simulink model "sv_power_control_subsystem_final"  (R2023b)
settings: Solver=FixedStepAuto  StartTime=0  StopTime=1  FixedStep=1/5e4/60  MaxStep=1e-4  RelTol=1e-4
StartFcn:
  | tic
StopFcn:
  | toc
undefined symbols (not defined in the file): Ion, Lithium
libraries: spsBatteryLib x30, simulink x30, spsIdealSwitchLib x30, spsSeriesRLCBranchLib x2, spsControlledCurrentSourceLib x1, spsGroundLib x1, spsTriangleGeneratorLib x1, spsVoltageMeasurementLib x1, spspowerguiLib x1
settings Model: SimulationMode=accelerator  Creator=The MathWorks, Inc.  LastModifiedBy=zhaoxu
settings SolverCC: ZeroCrossAlgorithm=Adaptive  AlgebraicLoopSolver=TrustRegion  AutoInsertRateTranBlk=on
settings DataIOCC: LimitDataPoints=on  SaveFormat=Array  SaveOutput=off  SignalLogging=off  SaveTime=off  ReturnWorkspaceOutputs=off
settings OptimizationCC: ExpressionDepthLimit=2147483647  LifeSpan=inf
settings DebuggingCC: UnderspecifiedInitializationDetection=Classic  MergeDetectMultiDrivingBlocksExec=none  IgnoredZcDiagnostic=none  SolverPrmCheckMsg=warning  MultiTaskRateTransMsg=warning  FcnCallInpInsideContextMsg=warning  UnconnectedInputMsg=warning  UnconnectedOutputMsg=warning  UnconnectedLineMsg=warning  StateNameClashWarn=warning  SFUnexpectedBacktrackingDiag=warning  SFNoUnconditionalDefaultTransitionDiag=warning  SFExecutionAtInitializationDiag=none  ArithmeticOperatorsInVariantConditions=warning
settings HardwareCC: ProdHWDeviceType=AMD->x86-64 (Windows64)
settings ModelReferenceCC: EnableRefExpFcnMdlSchedulingChecks=on  PropagateSignalLabelsOutOfModel=off
settings SFSimCC: SimUseLocalCustomCode=off  CustomCodeUndefinedFunction=UseInterfaceOnly  SimTargetLang=C++
settings RTWCC: RTWUseLocalCustomCode=off  DLArmComputeVersion=19.05
settings CodeAppCC: StateflowObjectComments=on
settings GRTTargetCC: TargetLangStandard=C89/C90 (ANSI)  CombineOutputUpdateFcns=off  GRTInterface=on
settings ConfigComp: CovMetricSettings=dw  CovSaveCumulativeToWorkspaceVar=on  CovSaveSingleToWorkspaceVar=on  CovExternalEMLEnable=off  CovSFcnEnable=off
settings SimscapeCC: SimscapeNormalizeSystem=off  SimscapeNominalValues={1, 'bar'; 1, 'cm^3/s'; 1, 'bar*kg/s'; 1, 'kJ/kg'; 1, 'kW'; }

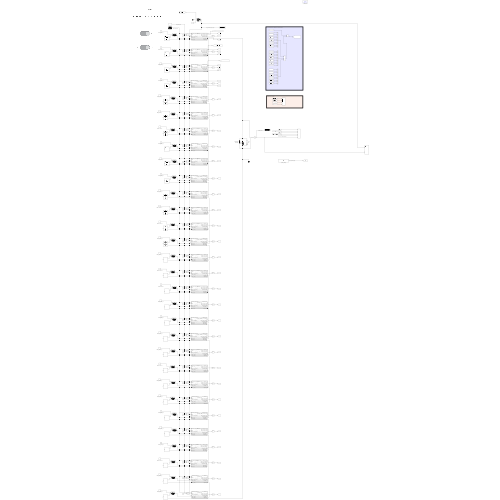
[thumbnail: Simulink's stored preview of the top-level diagram]
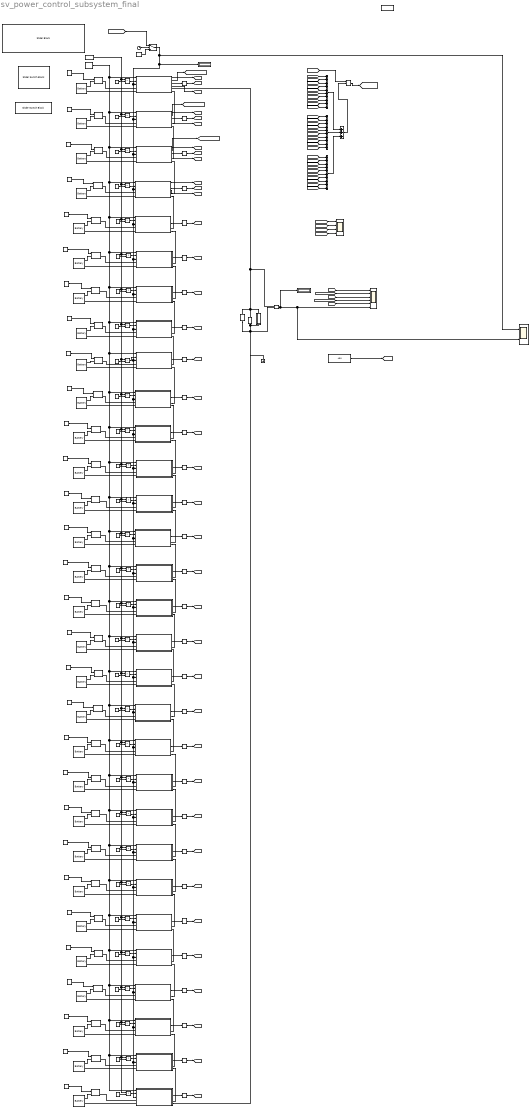
== system sv_power_control_subsystem_final ==
  note: Synchronous_PWM
  note: The average given voltage for each module
  Add1 : Sum  Inputs=+++
  Add2 : Sum  Inputs=++++++++++
  Add3 : Sum  Inputs=++++++++++
  Add4 : Sum  Inputs=++++++++++
  Battery{1..30} (30 alike) : spsBatteryLib/Battery  BatType=Lithium-Ion  ShowTempParam=off  ThermalPreset=no  ShowAgeParam=off  NomV=25.6  NomQ=50  SOC=70  Batt_Tr=30  PresetModel=on  MaxQ=50  MinV=19.2  FullV=29.7981  Dis_rate=21.7391  R=0.00512  Normal_OP=45.2174  expZone="[27.6579      2.45652]"  current=[6.5 13 32.5]  Units=Ampere-hour  Tci=20  NomT=20  T2=-30  MaxQ2=4.8  FullV2=7.1  Normal_OP2=5.655  expZone2="[6.58           1]"  Rca=0.6  ti=2000  Dp=0  Neq0=0  Tsim=1e6  Ta1=25  Qeol=5.4*0.9  Reol=0.013333*1.2  Char_age=[2.3478, 3]  Dis_age=[2.3478, 10]  N1=1500  N2=10500  N3=1000  N4=1400  Ta2=45  N5=950
  Battery_Enable_{1..30} (30 alike) : Constant
  Clock : Clock
  Compare To Constant{,1..29} (30 alike) : simulink/Logic and Bit Operations/Compare To Constant  relop=>=  const=15  OutDataTypeStr=uint8
  Constant : Constant  Value=10
  Constant1 : Constant  Value=0
  Constant10 : Constant  Value=8
  Constant11 : Constant  Value=9
  Constant12 : Constant  Value=10
  Constant13 : Constant  Value=11
  Constant14 : Constant  Value=12
  Constant15 : Constant  Value=17
  Constant16 : Constant  Value=18
  Constant17 : Constant  Value=19
  Constant18 : Constant  Value=20
  Constant19 : Constant  Value=21
  Constant2 : Constant
  Constant20 : Constant  Value=13
  Constant21 : Constant  Value=14
  Constant22 : Constant  Value=15
  Constant23 : Constant  Value=16
  Constant24 : Constant  Value=25
  Constant25 : Constant  Value=26
  Constant26 : Constant  Value=27
  Constant27 : Constant  Value=28
  Constant28 : Constant  Value=29
  Constant29 : Constant  Value=22
  Constant3 : Constant  Value=2
  Constant30 : Constant  Value=23
  Constant31 : Constant  Value=24
  Constant4 : Constant  Value=3
  Constant5 : Constant  Value=4
  Constant6 : Constant  Value=5
  Constant7 : Constant  Value=1/5e4/30
  Constant8 : Constant  Value=6
  Constant9 : Constant  Value=7
  Cyclic load : Subsystem
  Display : Display
  Display2 : Display
  Divide : Product  Inputs=*/
  Fixed load : spsSeriesRLCBranchLib/Series RLC Branch  LConnTagsString=__new0  RConnTagsString=__new0  BranchType=R  Resistance=3.75  Inductance=1e-3  SetiL0=off  InitialCurrent=0  Capacitance=1e-6  Setx0=off  InitialVoltage=0  Measurements=None
  Ground : spsGroundLib/Ground  LConnTagsString=a
  Ideal Switch{,1..29} (30 alike) : spsIdealSwitchLib/Ideal Switch  Ron=0.001  Lon=0  IC=0  Rs=1e5  Cs=inf  Measurements=on
  Product{,1..29} (30 alike) : Product
  Scope : Scope  NumInputPorts=6
  Scope2 : Scope  NumInputPorts=4
  Scope3 : Scope  NumInputPorts=2
  Slider : SliderBlock  ScaleMin=400  ScaleMax=768
  Slider Switch : SliderSwitchBlock
      settings: Values={{'Off', 'On'}, [0 1]}
  Slider Switch1 : SliderSwitchBlock
      settings: Values={{'Off', 'On'}, [0 1]}
  Smoothing capacitor : spsSeriesRLCBranchLib/Series RLC Branch  LConnTagsString=__new0  RConnTagsString=__new0  BranchType=C  Resistance=1  Inductance=1e-3  SetiL0=off  InitialCurrent=0  Capacitance=1.6e-5  Setx0=off  InitialVoltage=0  Measurements=None
  Subsystem{,1..29} (30 alike) : Subsystem  ReferencedSubsystem=Subsystem_final
  Switch : Switch  Criteria=u2 > Threshold  Threshold=0.001  SaturateOnIntegerOverflow=off  InputSameDT=off
  System_Voltage : Constant  Value=450
  Triangle Generator : spsTriangleGeneratorLib/Triangle Generator  Freq=50000  Phase=0  Ts=0
  Voltage Measurement : spsVoltageMeasurementLib/Voltage Measurement  PhasorSimulation=off  OutputType=Complex  PSBequivalent=0
  powergui : spspowerguiLib/powergui  Priority=1  SimulationMode=Discrete  SampleTime=1/5e4/60  frequency=60  Iterations=50  frequencyindice=0  Pbase=100e6  ErrMax=1e-4  UnitsV=kV  UnitsW=MW  buscounter=0  FunctionMessages=off  echomessages=off  EnableUseOfTLC=off  CurrentSourceSwitches=off  DisableSnubberDevices=off  DisableRonSwitches=off  DisableVfSwitches=off  DisplayEquations=off  AutomaticDiscreteSolvers=off  SolverType=Tustin/Backward Euler (TBE)  Interpol=off  ExternalGateDelay=off  methode=off  Ts=100  x0status=blocks  SPID=on  SwTol=0  HookPort=off  NonlinearTolerance=1e-4  nMaxIteration=100  ContinueOnMaxIteration=off  RestoreLinks=warning  ResistiveCurrentMeasurement=off  Frange=[0:2:500]  Ylog=off  Xlog=on  ShowGrid=off  save=off  variable=ZData  structure=0  ZoomFFT=on  StartTime=0.0  cycles=1  DisplayStyle=1  fundamental=60  FreqAxis=off  MaxFrequency=1000  frequencyindicesteady=1  RmsSteady=1  display=off
  wires:
  Battery_Enable_1/1 -> Ideal Switch/1
  Battery_Enable_2/1 -> Ideal Switch1/1
  Battery_Enable_3/1 -> Ideal Switch2/1
  Battery_Enable_4/1 -> Ideal Switch3/1
  Battery_Enable_5/1 -> Ideal Switch4/1
  Battery_Enable_7/1 -> Ideal Switch6/1
  Battery_Enable_6/1 -> Ideal Switch5/1
  Subsystem1/3 -> Compare To Constant2/1
  Subsystem2/3 -> Compare To Constant3/1
  Subsystem4/3 -> Compare To Constant1/1
  Add1/1 -> Divide/2
  Subsystem/3 -> Compare To Constant/1
  Subsystem6/3 -> Compare To Constant4/1
  Subsystem3/3 -> Compare To Constant5/1
  Subsystem5/3 -> Compare To Constant6/1
  Product/1 -> Subsystem/2
  Product1/1 -> Subsystem4/2
  Product2/1 -> Subsystem1/2
  Product3/1 -> Subsystem2/2
  Product4/1 -> Subsystem6/2
  Product5/1 -> Subsystem3/2
  Product6/1 -> Subsystem5/2
  Constant1/1 -> Product/2
  Constant2/1 -> Product1/2
  Constant3/1 -> Product2/2
  Constant4/1 -> Product3/2
  Constant5/1 -> Product4/2
  Constant6/1 -> Product5/2
  Constant8/1 -> Product6/2
  Constant/1 -> Switch/3
  Clock/1 -> Switch/2
  [control_V] -> Divide/1
  Subsystem/1 -> [CV1]  "CV1"
  [CV1] -> Scope/1
  [Battery_Current_1] -> Scope/2
  [Battery_Current_2] -> Scope/4
  Subsystem4/1 -> [CV2]  "CV2"
  Subsystem1/1 -> [CV3]  "CV3"
  Subsystem2/1 -> [CV4]  "CV4"
  [CV2] -> Scope/3
  [i_load] -> Scope/5  "yclic load current"
  Compare To Constant/1 -> [BV1]
  Compare To Constant1/1 -> [BV2]
  Compare To Constant2/1 -> [BV3]
  Compare To Constant3/1 -> [BV4]
  Compare To Constant4/1 -> [BV5]
  Compare To Constant5/1 -> [BV6]
  Compare To Constant6/1 -> [BV7]
  Divide/1 -> [Average_voltage]
  [Average_voltage] -> Switch/1
  Subsystem/4 -> [S_PWM1]
  Subsystem4/4 -> [S_PWM2]
  Subsystem1/4 -> [S_PWM3]
  Subsystem2/4 -> [S_PWM4]
  [S_PWM1] -> Scope2/1
  [S_PWM2] -> Scope2/2
  [S_PWM3] -> Scope2/3
  [S_PWM4] -> Scope2/4
  Voltage Measurement/1 -> Scope3/2, Scope/6, Display2/1  "HV_BUS_Voltage"
  Product9/1 -> Subsystem8/2
  Constant14/1 -> Product12/2
  Constant12/1 -> Product10/2
  Constant9/1 -> Product7/2
  Compare To Constant9/1 -> [BV10]
  Subsystem10/3 -> Compare To Constant7/1
  Compare To Constant12/1 -> [BV13]
  Subsystem12/3 -> Compare To Constant10/1
  Battery_Enable_8/1 -> Ideal Switch7/1
  Compare To Constant8/1 -> [BV9]
  Constant13/1 -> Product11/2
  Compare To Constant10/1 -> [BV11]
  Battery_Enable_12/1 -> Ideal Switch11/1
  Product12/1 -> Subsystem11/2
  Subsystem11/3 -> Compare To Constant12/1
  Product8/1 -> Subsystem7/2
  Subsystem8/3 -> Compare To Constant9/1
  Subsystem7/3 -> Compare To Constant8/1
  Product7/1 -> Subsystem10/2
  Product11/1 -> Subsystem9/2
  Battery_Enable_11/1 -> Ideal Switch10/1
  Constant10/1 -> Product8/2
  Constant11/1 -> Product9/2
  Battery_Enable_13/1 -> Ideal Switch12/1
  Compare To Constant7/1 -> [BV8]
  Compare To Constant11/1 -> [BV12]
  Product10/1 -> Subsystem12/2
  Battery_Enable_9/1 -> Ideal Switch8/1
  Subsystem9/3 -> Compare To Constant11/1
  Battery_Enable_10/1 -> Ideal Switch9/1
  Constant16/1 -> Product21/2
  Product13/1 -> Subsystem15/2
  Constant15/1 -> Product20/2
  Compare To Constant19/1 -> [BV17]
  Battery_Enable_14/1 -> Ideal Switch21/1
  Battery_Enable_17/1 -> Ideal Switch15/1
  Product14/1 -> Subsystem21/2
  Battery_Enable_22/1 -> Ideal Switch20/1
  Subsystem21/3 -> Compare To Constant14/1
  Battery_Enable_15/1 -> Ideal Switch13/1
  Product15/1 -> Subsystem14/2
  Subsystem14/3 -> Compare To Constant15/1
  Product19/1 -> Subsystem13/2
  Constant18/1 -> Product14/2
  Compare To Constant14/1 -> [BV21]
  Product20/1 -> Subsystem19/2
  Subsystem19/3 -> Compare To Constant20/1
  Compare To Constant13/1 -> [BV20]
  Compare To Constant20/1 -> [BV18]
  Compare To Constant15/1 -> [BV22]
  Subsystem15/3 -> Compare To Constant13/1
  Battery_Enable_16/1 -> Ideal Switch14/1
  Constant17/1 -> Product13/2
  Compare To Constant21/1 -> [BV19]
  Constant19/1 -> Product15/2
  Product21/1 -> Subsystem20/2
  Constant23/1 -> Product19/2
  Subsystem20/3 -> Compare To Constant21/1
  Subsystem13/3 -> Compare To Constant19/1
  Constant20/1 -> Product16/2
  Compare To Constant18/1 -> [BV16]
  Subsystem18/3 -> Compare To Constant16/1
  Constant21/1 -> Product17/2
  Product16/1 -> Subsystem18/2
  Battery_Enable_21/1 -> Ideal Switch19/1
  Compare To Constant16/1 -> [BV14]
  Constant22/1 -> Product18/2
  Battery_Enable_19/1 -> Ideal Switch17/1
  Product18/1 -> Subsystem17/2
  Subsystem17/3 -> Compare To Constant18/1
  Product17/1 -> Subsystem16/2
  Subsystem16/3 -> Compare To Constant17/1
  Battery_Enable_18/1 -> Ideal Switch16/1
  Battery_Enable_20/1 -> Ideal Switch18/1
  Compare To Constant17/1 -> [BV15]
  Constant7/1 -> Product4/1, Product5/1, Product10/1, Product11/1, Product16/1, Product17/1, Product13/1, Product14/1, Product25/1, Product22/1, Product23/1, Product24/1, Product29/1, Product28/1, Product27/1, Product26/1, Product15/1, Product21/1, Product20/1, Product19/1, Product18/1, Product12/1, Product9/1, Product8/1, Product7/1, Product6/1, Product3/1, Product2/1, Product1/1, Product/1  "PWM_Phase_Base"
  Battery_Enable_28/1 -> Ideal Switch26/1
  Product25/1 -> Subsystem25/2
  Subsystem25/3 -> Compare To Constant25/1
  Compare To Constant25/1 -> [BV23]
  Subsystem26/3 -> Compare To Constant26/1
  Triangle Generator/1 -> Subsystem/1, Subsystem4/1, Subsystem1/1, Subsystem2/1, Subsystem6/1, Subsystem3/1, Subsystem10/1, Subsystem8/1, Subsystem12/1, Subsystem9/1, Subsystem18/1, Subsystem16/1, Subsystem13/1, Subsystem19/1, Subsystem20/1, Subsystem15/1, Subsystem21/1, Subsystem25/1, Subsystem22/1, Subsystem27/1, Subsystem28/1, Subsystem24/1, Subsystem29/1, Subsystem23/1, Subsystem26/1, Subsystem14/1, Subsystem17/1, Subsystem11/1, Subsystem7/1, Subsystem5/1  "PWM_Ref_Signal"
  Battery_Enable_27/1 -> Ideal Switch25/1
  Product26/1 -> Subsystem26/2
  Battery_Enable_29/1 -> Ideal Switch27/1
  Compare To Constant26/1 -> [BV24]
  Subsystem22/3 -> Compare To Constant27/1
  Subsystem28/3 -> Compare To Constant29/1
  Product29/1 -> Subsystem28/2
  Compare To Constant29/1 -> [BV27]
  Compare To Constant28/1 -> [BV26]
  Battery_Enable_30/1 -> Ideal Switch28/1
  Product27/1 -> Subsystem22/2
  Battery_Enable_25/1 -> Ideal Switch23/1
  Product23/1 -> Subsystem29/2
  Compare To Constant23/1 -> [BV29]
  Subsystem29/3 -> Compare To Constant23/1
  Battery_Enable_24/1 -> Ideal Switch22/1
  Subsystem23/3 -> Compare To Constant24/1
  Subsystem24/3 -> Compare To Constant22/1
  Constant24/1 -> Product28/2
  Constant26/1 -> Product22/2
  Product22/1 -> Subsystem24/2
  Constant29/1 -> Product25/2
  Battery_Enable_23/1 -> Ideal Switch29/1
  Constant28/1 -> Product24/2
  Product24/1 -> Subsystem23/2
  Constant27/1 -> Product23/2
  Compare To Constant22/1 -> [BV28]
  Battery_Enable_26/1 -> Ideal Switch24/1
  Subsystem27/3 -> Compare To Constant28/1
  Compare To Constant27/1 -> [BV25]
  Compare To Constant24/1 -> [BV30]
  Constant30/1 -> Product26/2
  Constant31/1 -> Product27/2
  Product28/1 -> Subsystem27/2
  Constant25/1 -> Product29/2
  [BV30] -> Add4/10
  [BV21] -> Add4/1
  [BV22] -> Add4/2
  [BV23] -> Add4/3
  [BV24] -> Add4/4
  [BV25] -> Add4/5
  [BV26] -> Add4/6
  [BV27] -> Add4/7
  [BV28] -> Add4/8
  [BV29] -> Add4/9
  [BV11] -> Add3/1
  [BV12] -> Add3/2
  [BV13] -> Add3/3
  [BV14] -> Add3/4
  [BV15] -> Add3/5
  [BV16] -> Add3/6
  [BV17] -> Add3/7
  [BV18] -> Add3/8
  [BV19] -> Add3/9
  [BV20] -> Add3/10
  [BV1] -> Add2/1
  [BV2] -> Add2/2
  [BV3] -> Add2/3
  [BV4] -> Add2/4
  [BV5] -> Add2/5
  [BV6] -> Add2/6
  [BV7] -> Add2/7
  [BV8] -> Add2/8
  [BV9] -> Add2/9
  [BV10] -> Add2/10
  Add4/1 -> Add1/3
  Add3/1 -> Add1/2
  Add2/1 -> Add1/1
  Switch/1 -> Scope3/1, Display/1, Subsystem23/3, Subsystem29/3, Subsystem24/3, Subsystem28/3, Subsystem27/3, Subsystem22/3, Subsystem26/3, Subsystem25/3, Subsystem14/3, Subsystem21/3, Subsystem15/3, Subsystem20/3, Subsystem19/3, Subsystem13/3, Subsystem17/3, Subsystem16/3, Subsystem18/3, Subsystem11/3, Subsystem9/3, Subsystem12/3, Subsystem8/3, Subsystem7/3, Subsystem10/3, Subsystem5/3, Subsystem3/3, Subsystem6/3, Subsystem2/3, Subsystem1/3, Subsystem4/3, Subsystem/3  "Single_Modular_Voltage_Target"
  System_Voltage/1 -> [control_V]  "Target_HV_BUS_Voltage"
  Subsystem/2 -> [Battery_Current_1]
  Subsystem4/2 -> [Battery_Current_2]
  Subsystem1/2 -> [Battery_Current_3]
  connections:
  Ideal Switch/LConn1 -- Battery1/LConn1
  Subsystem/LConn2 -- Battery1/LConn2
  Subsystem/LConn1 -- Ideal Switch/RConn1
  Fixed load/RConn1 -- Ground/LConn1 -- Subsystem23/RConn2 -- Smoothing capacitor/RConn1 -- Voltage Measurement/LConn2 -- Cyclic load/LConn1
  Subsystem4/LConn2 -- Battery2/LConn2
  Ideal Switch1/LConn1 -- Battery2/LConn1
  Subsystem4/LConn1 -- Ideal Switch1/RConn1
  Subsystem4/RConn1 -- Subsystem/RConn2
  Subsystem1/LConn2 -- Battery3/LConn2
  Subsystem1/LConn1 -- Ideal Switch2/RConn1
  Ideal Switch2/LConn1 -- Battery3/LConn1
  Subsystem1/RConn1 -- Subsystem4/RConn2
  Subsystem2/LConn2 -- Battery4/LConn2
  Subsystem2/LConn1 -- Ideal Switch3/RConn1
  Subsystem2/RConn1 -- Subsystem1/RConn2
  Ideal Switch3/LConn1 -- Battery4/LConn1
  Subsystem5/LConn1 -- Ideal Switch6/RConn1
  Ideal Switch6/LConn1 -- Battery7/LConn1
  Ideal Switch4/LConn1 -- Battery5/LConn1
  Subsystem3/LConn2 -- Battery6/LConn2
  Subsystem6/LConn1 -- Ideal Switch4/RConn1
  Subsystem3/LConn1 -- Ideal Switch5/RConn1
  Ideal Switch5/LConn1 -- Battery6/LConn1
  Subsystem5/LConn2 -- Battery7/LConn2
  Subsystem6/LConn2 -- Battery5/LConn2
  Subsystem2/RConn2 -- Subsystem6/RConn1
  Subsystem6/RConn2 -- Subsystem3/RConn1
  Subsystem3/RConn2 -- Subsystem5/RConn1
  Voltage Measurement/LConn1 -- Subsystem/RConn1 -- Smoothing capacitor/LConn1 -- Fixed load/LConn1 -- Cyclic load/RConn1
  Subsystem10/LConn1 -- Ideal Switch7/RConn1
  Ideal Switch12/LConn1 -- Battery13/LConn1
  Subsystem10/LConn2 -- Battery8/LConn2
  Subsystem7/RConn1 -- Subsystem10/RConn2
  Subsystem8/LConn1 -- Ideal Switch9/RConn1
  Subsystem5/RConn2 -- Subsystem10/RConn1
  Subsystem8/RConn2 -- Subsystem12/RConn1
  Subsystem7/LConn1 -- Ideal Switch8/RConn1
  Subsystem12/LConn1 -- Ideal Switch10/RConn1
  Subsystem12/LConn2 -- Battery11/LConn2
  Ideal Switch7/LConn1 -- Battery8/LConn1
  Subsystem11/LConn2 -- Battery13/LConn2
  Subsystem9/LConn1 -- Ideal Switch11/RConn1
  Subsystem8/RConn1 -- Subsystem7/RConn2
  Ideal Switch11/LConn1 -- Battery12/LConn1
  Ideal Switch9/LConn1 -- Battery10/LConn1
  Subsystem11/LConn1 -- Ideal Switch12/RConn1
  Ideal Switch10/LConn1 -- Battery11/LConn1
  Subsystem9/LConn2 -- Battery12/LConn2
  Subsystem7/LConn2 -- Battery9/LConn2
  Subsystem8/LConn2 -- Battery10/LConn2
  Subsystem9/RConn2 -- Subsystem11/RConn1
  Ideal Switch8/LConn1 -- Battery9/LConn1
  Subsystem12/RConn2 -- Subsystem9/RConn1
  Ideal Switch20/LConn1 -- Battery22/LConn1
  Subsystem21/RConn2 -- Subsystem14/RConn1
  Ideal Switch18/LConn1 -- Battery20/LConn1
  Subsystem16/LConn2 -- Battery19/LConn2
  Subsystem15/LConn1 -- Ideal Switch13/RConn1
  Subsystem14/LConn2 -- Battery17/LConn2
  Subsystem21/LConn2 -- Battery16/LConn2
  Ideal Switch21/LConn1 -- Battery14/LConn1
  Subsystem14/LConn1 -- Ideal Switch15/RConn1
  Subsystem13/LConn2 -- Battery21/LConn2
  Ideal Switch17/LConn1 -- Battery19/LConn1
  Subsystem17/RConn2 -- Subsystem13/RConn1
  Subsystem15/RConn2 -- Subsystem21/RConn1
  Ideal Switch13/LConn1 -- Battery15/LConn1
  Subsystem13/LConn1 -- Ideal Switch19/RConn1
  Subsystem19/RConn1 -- Subsystem13/RConn2
  Subsystem19/LConn2 -- Battery22/LConn2
  Ideal Switch19/LConn1 -- Battery21/LConn1
  Subsystem18/RConn2 -- Subsystem16/RConn1
  Subsystem20/RConn1 -- Subsystem19/RConn2
  Ideal Switch14/LConn1 -- Battery16/LConn1
  Subsystem11/RConn2 -- Subsystem18/RConn1
  Subsystem15/LConn2 -- Battery15/LConn2
  Subsystem18/LConn1 -- Ideal Switch16/RConn1
  Subsystem20/RConn2 -- Subsystem15/RConn1
  Subsystem17/LConn2 -- Battery20/LConn2
  Subsystem16/LConn1 -- Ideal Switch17/RConn1
  Subsystem21/LConn1 -- Ideal Switch14/RConn1
  Subsystem16/RConn2 -- Subsystem17/RConn1
  Subsystem19/LConn1 -- Ideal Switch20/RConn1
  Subsystem20/LConn1 -- Ideal Switch21/RConn1
  Subsystem17/LConn1 -- Ideal Switch18/RConn1
  Subsystem18/LConn2 -- Battery18/LConn2
  Ideal Switch16/LConn1 -- Battery18/LConn1
  Ideal Switch15/LConn1 -- Battery17/LConn1
  Subsystem20/LConn2 -- Battery14/LConn2
  Subsystem25/LConn1 -- Ideal Switch25/RConn1
  Subsystem27/RConn1 -- Subsystem22/RConn2
  Subsystem27/LConn1 -- Ideal Switch28/RConn1
  Subsystem28/RConn2 -- Subsystem24/RConn1
  Ideal Switch25/LConn1 -- Battery27/LConn1
  Subsystem28/LConn1 -- Ideal Switch29/RConn1
  Subsystem14/RConn2 -- Subsystem25/RConn1
  Subsystem28/RConn1 -- Subsystem27/RConn2
  Subsystem25/RConn2 -- Subsystem26/RConn1
  Ideal Switch23/LConn1 -- Battery25/LConn1
  Ideal Switch22/LConn1 -- Battery24/LConn1
  Subsystem24/RConn2 -- Subsystem29/RConn1
  Subsystem28/LConn2 -- Battery23/LConn2
  Ideal Switch28/LConn1 -- Battery30/LConn1
  Subsystem24/LConn1 -- Ideal Switch22/RConn1
  Subsystem29/RConn2 -- Subsystem23/RConn1
  Ideal Switch26/LConn1 -- Battery28/LConn1
  Subsystem29/LConn1 -- Ideal Switch23/RConn1
  Subsystem23/LConn1 -- Ideal Switch24/RConn1
  Subsystem24/LConn2 -- Battery24/LConn2
  Ideal Switch27/LConn1 -- Battery29/LConn1
  Ideal Switch29/LConn1 -- Battery23/LConn1
  Subsystem29/LConn2 -- Battery25/LConn2
  Subsystem26/LConn1 -- Ideal Switch26/RConn1
  Subsystem27/LConn2 -- Battery30/LConn2
  Subsystem25/LConn2 -- Battery27/LConn2
  Subsystem22/LConn1 -- Ideal Switch27/RConn1
  Subsystem26/LConn2 -- Battery28/LConn2
  Subsystem23/LConn2 -- Battery26/LConn2
  Subsystem26/RConn2 -- Subsystem22/RConn1
  Subsystem22/LConn2 -- Battery29/LConn2
  Ideal Switch24/LConn1 -- Battery26/LConn1

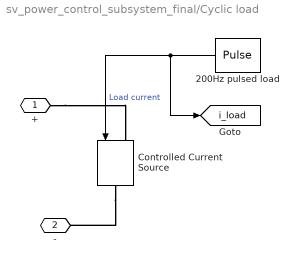
== system sv_power_control_subsystem_final/Cyclic load ==
  200Hz pulsed load : DiscretePulseGenerator  PulseType=Time based  Amplitude=2  Period=1/200  PulseWidth=50  PhaseDelay=1/400
  Controlled Current Source : spsControlledCurrentSourceLib/Controlled Current Source  Initialize=on  Source_Type=AC  Amplitude=0  Phase=0  Frequency=0  Measurements=None
  + : PMIOPort  Side=Right
  - : PMIOPort  Port=2  Side=Left
  tag scope: i_load=global
  wires:
  200Hz pulsed load/1 -> [i_load], Controlled Current Source/1  "Load current"
  connections:
  Controlled Current Source/RConn1 -- -/RConn1
  +/RConn1 -- Controlled Current Source/LConn1
